simulink model "test_signalGen"  (R2023b)
settings: Solver=FixedStepAuto  StartTime=0.0  StopTime=2.2  FixedStep=1/30  RelTol=1e-8
libraries: sensors_subsystems x1
settings Model: Creator=brent  LastModifiedBy=brent

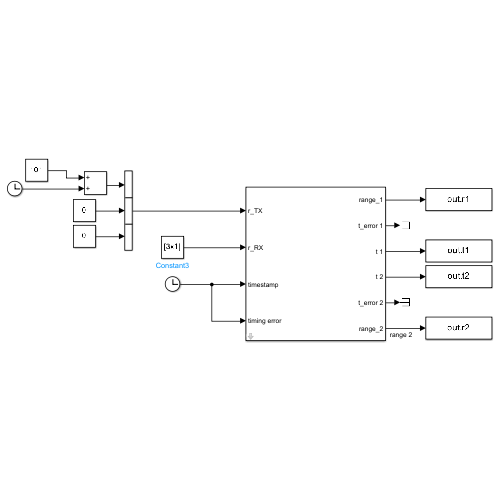
[thumbnail: Simulink's stored preview of the top-level diagram]
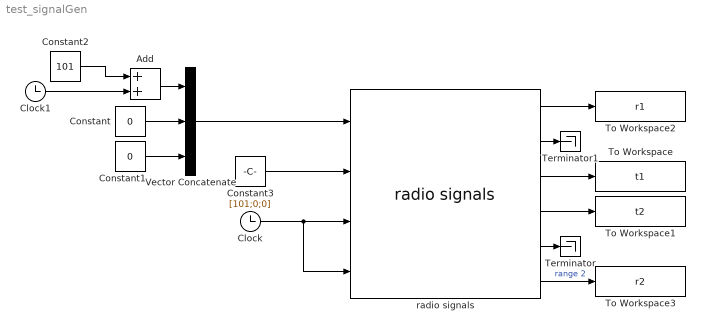
== system test_signalGen ==
  Add : Sum
  Clock : Clock
  Clock1 : Clock
  Constant : Constant  Value=0
  Constant1 : Constant  Value=0
  Constant2 : Constant  Value=101
  Constant3 : Constant  Value=[101;0;0]
  Terminator : Terminator
  Terminator1 : Terminator
  To Workspace : ToWorkspace  VariableName=t1  SaveFormat=Timeseries  SampleTime=-1
      settings: Save2DSignal=2-D array (concatenate along first dimension)
  To Workspace1 : ToWorkspace  VariableName=t2  SaveFormat=Timeseries  SampleTime=-1
      settings: Save2DSignal=2-D array (concatenate along first dimension)
  To Workspace2 : ToWorkspace  VariableName=r1  SaveFormat=Timeseries  SampleTime=-1
      settings: Save2DSignal=2-D array (concatenate along first dimension)
  To Workspace3 : ToWorkspace  VariableName=r2  SaveFormat=Timeseries  SampleTime=-1
      settings: Save2DSignal=2-D array (concatenate along first dimension)
  Vector Concatenate : Concatenate  NumInputs=3
  radio signals : sensors_subsystems/radio signals  light_speed=Inf  R_m=100  sampleTime=0.1  delay=1  pulseSamples=10  pulseWidth=1
      settings: SourceProductName=Sensors library
  wires:
  Vector Concatenate/1 -> radio signals/1
  Constant3/1 -> radio signals/2
  Clock/1 -> radio signals/4, radio signals/3
  Constant1/1 -> Vector Concatenate/3
  Constant/1 -> Vector Concatenate/2
  Clock1/1 -> Add/2
  Constant2/1 -> Add/1
  Add/1 -> Vector Concatenate/1
  radio signals/1 -> To Workspace2/1
  radio signals/4 -> To Workspace1/1
  radio signals/6 -> To Workspace3/1  "range 2"
  radio signals/3 -> To Workspace/1
  radio signals/5 -> Terminator/1
  radio signals/2 -> Terminator1/1
